simulink model "send_a429"  (R2019b)
settings: Solver=FixedStepAuto  StartTime=0.0  StopTime=10.0  RelTol=1e-3
PreLoadFcn:
  | fprintf(1, '[PreLoadFcn] Load send_a429_sample_inputs.mat\n');
  | load send_a429_sample_inputs
model workspace (MAT data in the model file):
  ED247Configuration(1).name = 'T11M4_A429_SIMU2SWIM_BUS_1_350_10_I'
  ED247Configuration(1).direction = 'OUT'
  ED247Configuration(1).type = 'uint8'
  ED247Configuration(1).dimensions = 1
  ED247Configuration(1).width = 4
  ED247Configuration(1).size = 4
  ED247Configuration(1).sample_time = 1
  ED247Configuration(1).validity_duration = 1
  ED247Configuration(1).signal_type = 'A429'
  ED247Configuration(1).sample_size = 4
  ED247Configuration(2).name = 'T11M4_A429_SIMU2SWIM_BUS_1_200_10_I'
  ED247Configuration(2).direction = 'OUT'
  ED247Configuration(2).type = 'uint8'
  ED247Configuration(2).dimensions = 1
  ED247Configuration(2).width = 4
  ED247Configuration(2).size = 4
  ED247Configuration(2).sample_time = 1
  ED247Configuration(2).validity_duration = 1
  ED247Configuration(2).signal_type = 'A429'
  ED247Configuration(2).sample_size = 4
  ED247Configuration(3).name = 'T11M4_A429_SIMU2SWIM_BUS_1_200_11_I'
  ED247Configuration(3).direction = 'OUT'
  ED247Configuration(3).type = 'uint8'
  ED247Configuration(3).dimensions = 1
  ED247Configuration(3).width = 4
  ED247Configuration(3).size = 4
  ED247Configuration(3).sample_time = 1
  ED247Configuration(3).validity_duration = 1
  ED247Configuration(3).signal_type = 'A429'
  ED247Configuration(3).sample_size = 4
libraries: lib_ed247 x2
settings Model: Creator=odufour  LastModifiedBy=odufour
settings DataIOCC: ExternalInput=ds  LoadExternalInput=on
settings OptimizationCC: DefaultParameterBehavior=Inlined  EnhancedBackFolding=on  PassReuseOutputArgsAs=Individual arguments  ZeroExternalMemoryAtStartup=off  ZeroInternalMemoryAtStartup=off  OptimizeBlockOrder=speed  DifferentSizesBufferReuse=on  OptimizationCustomize=off  EfficientTunableParamExpr=on
settings DebuggingCC: ParameterTunabilityLossMsg=error  ArithmeticOperatorsInVariantConditions=warning
settings SFSimCC: MATLABDynamicMemAlloc=off  CustomCodeUndefinedFunction=UseInterfaceOnly
settings RTWCC: SystemTargetFile=ert.tlc  GenCodeOnly=on  TemplateMakefile=ert_default_tmf  GenerateReport=on  IncludeHyperlinkInReport=on  GenerateTraceInfo=on  GenerateTraceReport=on  GenerateTraceReportSl=on  GenerateTraceReportSf=on  GenerateTraceReportEml=on
settings CodeAppCC: ForceParamTrailComments=on  IgnoreCustomStorageClasses=off  OperatorAnnotations=on  SimulinkDataObjDesc=on  SFDataObjDesc=on  InsertBlockDesc=on
settings ERTTargetCC: TargetLangStandard=C99 (ISO)  GenerateSampleERTMain=on  InlinedParameterPlacement=NonHierarchical  ERTCustomFileTemplate=example_file_process.tlc

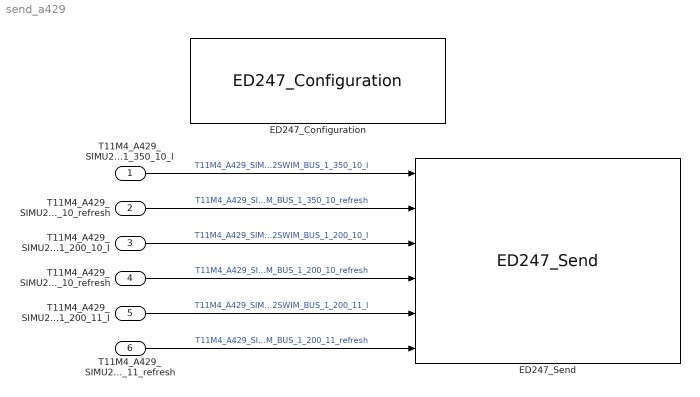
== system send_a429 ==
  T11M4_A429_SIMU2SWIM_BUS_1_350_10_I : Inport  OutDataTypeStr=uint8  PortDimensions=4  SampleTime=0.1
  T11M4_A429_SIMU2SWIM_BUS_1_350_10_refresh : Inport  Port=2  OutDataTypeStr=boolean
  T11M4_A429_SIMU2SWIM_BUS_1_200_10_I : Inport  Port=3  OutDataTypeStr=uint8  PortDimensions=4  SampleTime=0.1
  T11M4_A429_SIMU2SWIM_BUS_1_200_10_refresh : Inport  Port=4  OutDataTypeStr=boolean
  T11M4_A429_SIMU2SWIM_BUS_1_200_11_I : Inport  Port=5  OutDataTypeStr=uint8  PortDimensions=4  SampleTime=0.1
  T11M4_A429_SIMU2SWIM_BUS_1_200_11_refresh : Inport  Port=6  OutDataTypeStr=boolean
  ED247_Configuration : lib_ed247/ED247_Configuration  configurationFilename='ecic_func_exchange_a429_uc_main_simple.xml'  enableLog=off  logFilename=''
      settings: SourceProductName=Airbus ED247
  ED247_Send : lib_ed247/ED247_Send  enable_refresh=on  show_port_labels=on
      settings: SourceProductName=Airbus ED247
  wires:
  T11M4_A429_SIMU2SWIM_BUS_1_350_10_I/1 -> ED247_Send/1  "T11M4_A429_SIMU2SWIM_BUS_1_350_10_I"
  T11M4_A429_SIMU2SWIM_BUS_1_200_10_I/1 -> ED247_Send/3  "T11M4_A429_SIMU2SWIM_BUS_1_200_10_I"
  T11M4_A429_SIMU2SWIM_BUS_1_200_11_I/1 -> ED247_Send/5  "T11M4_A429_SIMU2SWIM_BUS_1_200_11_I"
  T11M4_A429_SIMU2SWIM_BUS_1_350_10_refresh/1 -> ED247_Send/2  "T11M4_A429_SIMU2SWIM_BUS_1_350_10_refresh"
  T11M4_A429_SIMU2SWIM_BUS_1_200_10_refresh/1 -> ED247_Send/4  "T11M4_A429_SIMU2SWIM_BUS_1_200_10_refresh"
  T11M4_A429_SIMU2SWIM_BUS_1_200_11_refresh/1 -> ED247_Send/6  "T11M4_A429_SIMU2SWIM_BUS_1_200_11_refresh"
